simulink model "PROJECTQ2"  (R2022a)
settings: Solver=VariableStepAuto  StartTime=0.0  StopTime=10.0  RelTol=1e-3
settings Model: Creator=1234567890  LastModifiedBy=1234567890

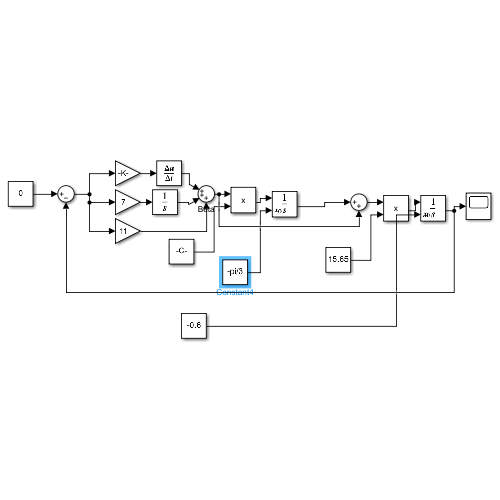
[thumbnail: Simulink's stored preview of the top-level diagram]
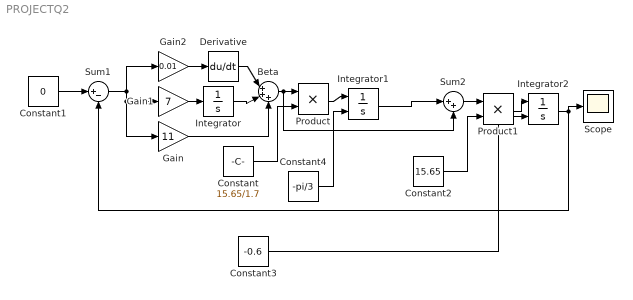
== system PROJECTQ2 ==
  Beta : Sum  Inputs=|+++
  Constant : Constant  Value=15.65/1.7
  Constant1 : Constant  Value=0
  Constant2 : Constant  Value=15.65
  Constant3 : Constant  Value=-0.6
  Constant4 : Constant  Value=-pi/3
  Derivative : Derivative
  Gain : Gain  Gain=11
  Gain1 : Gain  Gain=7
  Gain2 : Gain  Gain=0.01
  Integrator : Integrator
  Integrator1 : Integrator  InitialConditionSource=external
  Integrator2 : Integrator  InitialConditionSource=external
  Product : Product
  Product1 : Product
  Scope : Scope
  Sum1 : Sum  Inputs=|+-
  Sum2 : Sum  Inputs=|++
  wires:
  Sum1/1 -> Gain2/1, Gain1/1, Gain/1
  Constant1/1 -> Sum1/1
  Derivative/1 -> Beta/1
  Integrator/1 -> Beta/2
  Gain/1 -> Beta/3
  Gain1/1 -> Integrator/1
  Gain2/1 -> Derivative/1
  Beta/1 -> Sum2/2, Product/1
  Product/1 -> Integrator1/1
  Constant/1 -> Product/2
  Integrator1/1 -> Sum2/1
  Sum2/1 -> Product1/1
  Integrator2/1 -> Scope/1, Sum1/2
  Product1/1 -> Integrator2/1
  Constant2/1 -> Product1/2
  Constant3/1 -> Integrator2/2
  Constant4/1 -> Integrator1/2
